simulink model "W08_S1"  (R2024b)
settings: Solver=ode4  StartTime=0  StopTime=T_final  FixedStep=h  RelTol=1e-3
undefined symbols (not defined in the file or in its folder): beta_c, e_min, h, hand_over, k_neg, k_pos, Kd, Kd_x, Ki_x, Kp, Kp_x, mp, N_max, psi_fix, R_arrive, rp, T_hold, T_max, T_min, V_c, vane, WP_E, WP_N, x0, X_ff, X_max, y_pont
settings Model: Creator=admin  LastModifiedBy=admin
settings DataIOCC: ReturnWorkspaceOutputs=off

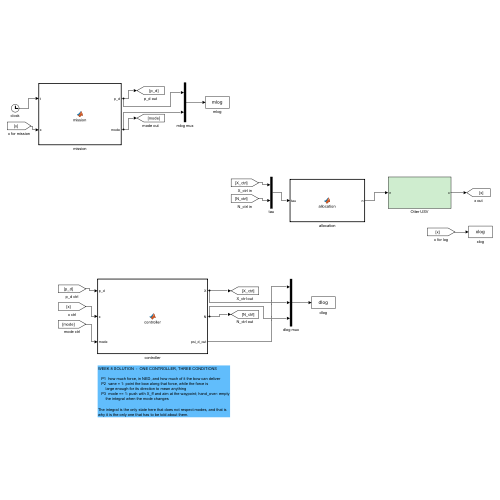
[thumbnail: Simulink's stored preview of the top-level diagram]
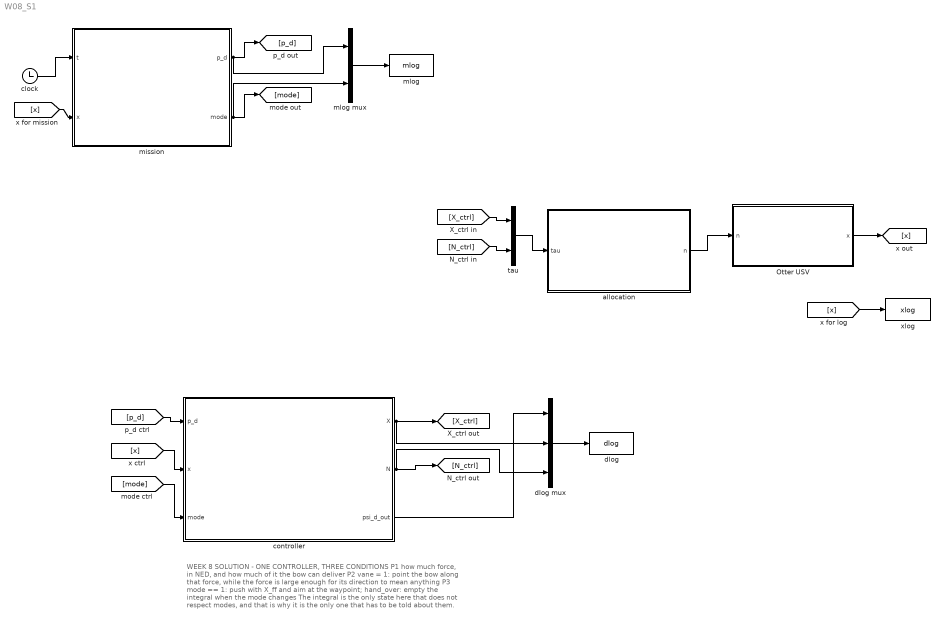
== system W08_S1 ==
  note: WEEK 8 SOLUTION  -  ONE CONTROLLER, THREE CONDITIONS
      |
      |    P1  how much force, in NED, and how much of it the bow can deliver
      |    P2  vane = 1: point the bow along that force, while the force is
      |        large enough for its direction to mean anything
      |    P3  mode == 1: push with X_ff and aim at the waypoint; hand_over: empty
      |        the integral when the mode changes
      |
      | The integral is the only state here that does not respect modes, and that is
      | why it is the only one that has to be told about them.
  Otter USV : Subsystem
  allocation : MATLAB Function  TreatAsAtomicUnit=on
  clock : Clock
  controller : MATLAB Function  TreatAsAtomicUnit=on
  dlog : ToWorkspace  VariableName=dlog  SaveFormat=Structure With Time  SampleTime=-1
  dlog mux : Mux  Inputs=3
  mission : MATLAB Function  TreatAsAtomicUnit=on
  mlog : ToWorkspace  VariableName=mlog  SaveFormat=Structure With Time  SampleTime=-1
  mlog mux : Mux  Inputs=2
  tau : Mux  Inputs=2
  xlog : ToWorkspace  VariableName=xlog  SaveFormat=Structure With Time  SampleTime=-1
  wires:
  clock/1 -> mission/1(t)
  [x] -> mission/2(x)
  mission/1(p_d) -> [p_d], mlog mux/1
  mission/2(mode) -> [mode], mlog mux/2
  mlog mux/1 -> mlog/1
  [X_ctrl] -> tau/1
  [N_ctrl] -> tau/2
  tau/1 -> allocation/1(tau)
  allocation/1(n) -> Otter USV/1(n)
  Otter USV/1(x) -> [x]
  [x] -> xlog/1
  [p_d] -> controller/1(p_d)
  [x] -> controller/2(x)
  [mode] -> controller/3(mode)
  controller/1(X) -> [X_ctrl], dlog mux/2
  controller/2(N) -> [N_ctrl], dlog mux/3
  controller/3(psi_d_out) -> dlog mux/1
  dlog mux/1 -> dlog/1

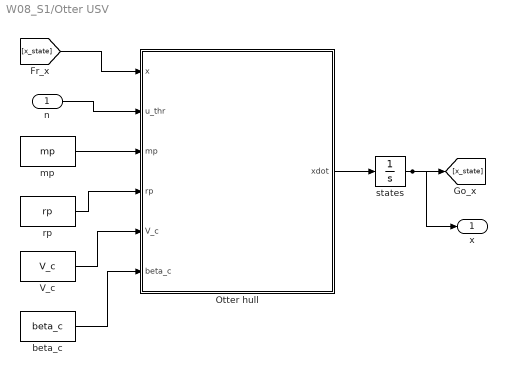
== system W08_S1/Otter USV ==
  n : Inport
  Otter hull : MATLAB Function  TreatAsAtomicUnit=on
  V_c : Constant  Value=V_c
  beta_c : Constant  Value=beta_c
  mp : Constant  Value=mp
  rp : Constant  Value=rp
  states : Integrator  InitialCondition=x0
  x : Outport
  wires:
  [x_state] -> Otter hull/1(x)
  rp/1 -> Otter hull/4(rp)
  n/1 -> Otter hull/2(u_thr)
  V_c/1 -> Otter hull/5(V_c)
  mp/1 -> Otter hull/3(mp)
  Otter hull/1(xdot) -> states/1
  beta_c/1 -> Otter hull/6(beta_c)
  states/1 -> [x_state], x/1

== matlab function W08_S1/allocation ==
  data: tau input; n output double size=[2 1]; y_pont parameter; k_pos parameter; k_neg parameter; T_max parameter; T_min parameter
function n = allocation(tau, y_pont, k_pos, k_neg, T_max, T_min)
%#codegen
%  6주차의 배분 그대로 / the allocation of Week 6, unchanged
T1 = tau(1)/2 + tau(2)/(2*y_pont);
T2 = tau(1)/2 - tau(2)/(2*y_pont);
s = 1;
if T1 > T_max, s = min(s, T_max/T1); end
if T2 > T_max, s = min(s, T_max/T2); end
if T1 < T_min, s = min(s, T_min/T1); end
if T2 < T_min, s = min(s, T_min/T2); end
T1 = s*T1;  T2 = s*T2;
k1 = k_pos;  if T1 < 0, k1 = k_neg; end
k2 = k_pos;  if T2 < 0, k2 = k_neg; end
n = [sign(T1)*sqrt(abs(T1)/k1); sign(T2)*sqrt(abs(T2)/k2)];

== matlab function W08_S1/mission ==
  settings: updateMethod=DISCRETE  sampleTime=h
  data: t input; p_d output double size=[2 1]; x input; mode output; WP_N parameter; WP_E parameter; R_arrive parameter; T_hold parameter; h parameter
function [p_d, mode] = mission(t, x, WP_N, WP_E, R_arrive, T_hold, h)
%#codegen
%MISSION  8주차 §8-5 의 상태기계. 규칙은 둘뿐이다.
%         The state machine of Week 8 §8-5: two rules only.
%
%    이동 중이고 목표에 R_arrive 안으로 들어오면  -> 유지, 시계를 0 으로
%    유지 중이고 T_hold 가 지나면                -> 다음 지점, 이동으로
%
%    in transit and inside R_arrive  -> hold, and reset the clock
%    in hold and T_hold has passed   -> the next waypoint, and transit
%
%  웨이포인트가 하나뿐이면 배는 처음부터 유지 모드에 있고 거기 머문다 —
%  1·2번 문제가 원하는 것이 그것이다.
%  With a single waypoint the vessel starts in hold and stays there, which is
%  what Problems 1 and 2 want.
persistent k mode_ held
if isempty(k), k = 1; mode_ = 1; held = 0; end
d = hypot(WP_N(k) - x(7), WP_E(k) - x(8));
if mode_ == 1 && d < R_arrive
    mode_ = 2;  held = 0;
elseif mode_ == 2
    held = held + h;
    if held >= T_hold
        if k < numel(WP_N), k = k + 1;  mode_ = 1;  else, mode_ = 3; end
    end
end
p_d  = [WP_N(k); WP_E(k)];
mode = mode_;

== matlab function W08_S1/Otter USV/Otter hull ==
  data: x input; xdot output double size=[12 1]; u_thr input; mp input; rp input; V_c input; beta_c input
function xdot = otter_hull(x, u_thr, mp, rp, V_c, beta_c)
% Fossen's otter.m, called unchanged from Tools/MSS/VESSELS.
%
%   x       12 states, fed back from the integrator
%   u_thr   propeller shaft speeds [rad/s]
%
% otter.m is not written for code generation, so the call is extrinsic and
% xdot has to be pre-sized for Simulink to know the output width.
coder.extrinsic('otter');

xdot = zeros(12,1);
xdot = otter(x, u_thr, mp, rp, V_c, beta_c);
end

== matlab function W08_S1/controller ==
  settings: updateMethod=DISCRETE  sampleTime=h
  data: p_d input; X output double size=[1 1]; x input; mode input; N output; psi_d_out output; Kp_x parameter; Ki_x parameter; Kd_x parameter; e_min parameter; X_max parameter; Kp parameter; Kd parameter; N_max parameter; psi_fix parameter; vane parameter; X_ff parameter; hand_over parameter; h parameter
function [X, N, psi_d_out] = controller(p_d, x, mode, Kp_x, Ki_x, Kd_x, e_min, X_max, Kp, Kd, N_max, psi_fix, vane, X_ff, hand_over, h)
%#codegen
%CONTROLLER  세 문제가 한 블록에 / all three problems, in one block.
psi = x(12);  u = x(1);  v = x(2);  r = x(6);
persistent In Ie
if isempty(In), In = 0;  Ie = 0; end
%
%  ── 문제 1a) 얼마의 힘이 어느 방향으로 / how much force, and where ────
%     위치 오차에 대한 PID 를 **북·동 두 방향 모두**에 대해 쓴다. 나오는 것은
%     추진기 이야기가 아니라 "이만큼의 힘이 이 방향으로 필요하다" 는 벡터다.
%     A PID on the position error, in both north and east. What comes out is
%     not yet a thruster: it is a vector saying how much force is wanted and
%     in which direction.
e_n = p_d(1) - x(7);  e_e = p_d(2) - x(8);
v_n = u*cos(psi) - v*sin(psi);        % 속도를 NED 로 / the velocity in NED
v_e = u*sin(psi) + v*cos(psi);
f_n = Kp_x*e_n + In - Kd_x*v_n;
f_e = Kp_x*e_e + Ie - Kd_x*v_e;
f   = hypot(f_n, f_e);
%
%  ── 문제 2) 그 힘의 방향으로 뱃머리를 / point the bow along that force ─
%     이 선체가 낼 수 있는 힘은 뱃머리 방향뿐이다 (6주차 §6-3: B 의 둘째 행이 0).
%     그러므로 필요한 힘 f 를 내려면 뱃머리가 f 를 향해야 한다. 조류가 밀면
%     적분이 상류 쪽 힘을 배우고, 뱃머리는 그것을 따라 조류에 맞선다.
%     The only force this hull can make points along its bow, so to deliver f
%     the bow must point along f. Under a current the integral learns an
%     upstream force and the bow follows it into the flow.
persistent psi_last
if isempty(psi_last), psi_last = psi; end
if vane ~= 0
    %  힘이 작으면 그 방향은 뜻을 잃는다 — 마지막 값을 붙들고 있는다.
    %  Too small a force has no meaningful direction: keep the last one.
    if f > e_min, psi_last = atan2(f_e, f_n); end
    psi_d = psi_last;
else
    %  문제 1: 선수각을 고정한다. f 가 뱃머리와 직각이면 한 뉴턴도 낼 수 없다.
    %  Problem 1 fixes the heading: when f lies across the bow, none of it
    %  can be made, and that is not the controller's fault.
    psi_d = psi_fix*pi/180;
end
%
%  ── 문제 3) 이동 중이면 / in transit ──────────────────────────────────
if mode == 1, psi_d = atan2(e_e, e_n); end
%
%  ── 문제 1b) 뱃머리 방향의 성분만 추진기로 / only the along-bow part ──
%     X 는 f 를 뱃머리에 정사영한 것이다. 옆 성분은 아무도 낼 수 없고,
%     그것이 1번 문제가 재는 양이다.
X = f_n*cos(psi) + f_e*sin(psi);
if mode == 1
    X = X_ff;                                   % 이동 중에는 일정한 추진력
    if hand_over ~= 0, In = 0;  Ie = 0; end     % 유지를 깨끗한 적분으로 시작
end
X = min(max(X, -X_max), X_max);
%  적분은 힘이 한계에 있지 않을 때만 쌓는다 (2주차 §2-11)
%  Integrate only while there is room — the anti-windup of Week 2
if abs(X) < X_max - 1e-9
    In = In + h*Ki_x*e_n;
    Ie = Ie + h*Ki_x*e_e;
end
%
%  ── 요 모멘트: 4주차의 오토파일럿 그대로 / the Week 4 autopilot ───────
ee = atan2(sin(psi_d - psi), cos(psi_d - psi));
N  = Kp*ee - Kd*r;
N  = min(max(N, -N_max), N_max);
if mode == 3, X = 0;  N = 0; end                % 끝 / done
psi_d_out = psi_d*180/pi;
